simulink model "twotanks_analitico"  (R2017a)
settings: Solver=FixedStepAuto  StartTime=0.0  StopTime=150  FixedStep=0.1  RelTol=1e-3
values from neighbouring files (symbols this model uses):
  H1 = (H1+H1')/2    [MPC_RODAR_PRIMEIRO.m]
  H2 = (H2+H2')/2    [MPC_RODAR_PRIMEIRO.m]
  Phi1 = [Phi1; sysi1.C*sysi1.A^(k)]    [MPC_RODAR_PRIMEIRO.m]
  Phi2 = [Phi2; sysi2.C*sysi2.A^(k)]    [MPC_RODAR_PRIMEIRO.m]
  Q1 = diag(repmat(q,1,Hp))    [MPC_RODAR_PRIMEIRO.m]
  Q2 = diag(repmat(q,1,Hp))    [MPC_RODAR_PRIMEIRO.m]
  Theta1 = [Theta1 aux1]    [MPC_RODAR_PRIMEIRO.m]
  Theta2 = [Theta2 aux2]    [MPC_RODAR_PRIMEIRO.m]
  Vd = 0.00001*eye(nx)    [MPC_RODAR_PRIMEIRO.m]
  Vn = 0.00001*eye(ny)    [MPC_RODAR_PRIMEIRO.m]
undefined symbols (not defined in the file or in its folder): sysi1, sysi2
libraries: simulink x2
settings Model: Creator=raonymaiafontes  LastModifiedBy=aguia
settings SolverCC: ZeroCrossAlgorithm=Adaptive
settings DebuggingCC: MaxConsecutiveZCsMsg=none

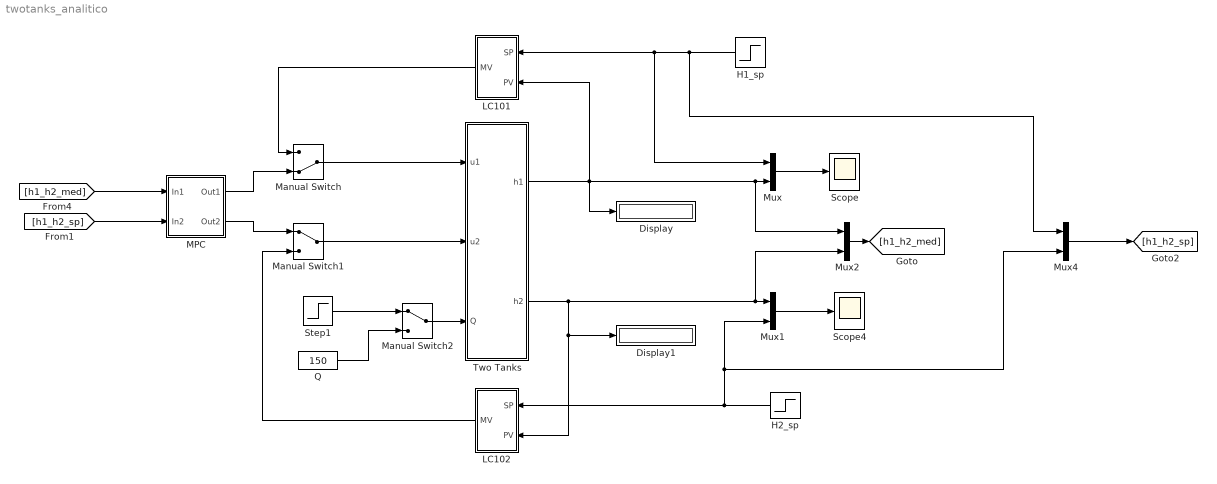
== system twotanks_analitico ==
  Display : Display
  Display1 : Display
  H1_sp : Step  Time=120  Before=0.65  After=0.35  SampleTime=0
  H2_sp : Step  Time=20  Before=0.28  After=0.678  SampleTime=0
  LC101 : Subsystem
  LC102 : Subsystem
  MPC : Subsystem
  Manual Switch : ManualSwitch  CurrentSetting=0
  Manual Switch1 : ManualSwitch
  Manual Switch2 : ManualSwitch
  Mux{,1..2,4} (4 alike) : Mux  Inputs=2
  Q : Constant  Value=150
  Scope : Scope
  Scope4 : Scope
  Step1 : Step  Time=70  Before=150  After=30  SampleTime=0
  Two Tanks : Subsystem
  wires:
  Manual Switch/1 -> Two Tanks/1(u1)
  LC101/1(MV) -> Manual Switch/1
  Manual Switch1/1 -> Two Tanks/2(u2)
  LC102/1(MV) -> Manual Switch1/2
  Manual Switch2/1 -> Two Tanks/3(Q)
  Step1/1 -> Manual Switch2/1
  Q/1 -> Manual Switch2/2
  Mux/1 -> Scope/1
  Mux1/1 -> Scope4/1
  Mux2/1 -> [h1_h2_med]
  Mux4/1 -> [h1_h2_sp]
  Two Tanks/1(h1) -> Mux2/1, Mux/2, LC101/2(PV), Display/1
  Two Tanks/2(h2) -> LC102/2(PV), Display1/1, Mux2/2, Mux1/1
  H2_sp/1 -> Mux4/2, Mux1/2, LC102/1(SP)
  H1_sp/1 -> Mux4/1, Mux/1, LC101/1(SP)
  [h1_h2_med] -> MPC/1(In1)
  [h1_h2_sp] -> MPC/2(In2)
  MPC/2(Out2) -> Manual Switch1/1
  MPC/1(Out1) -> Manual Switch/2

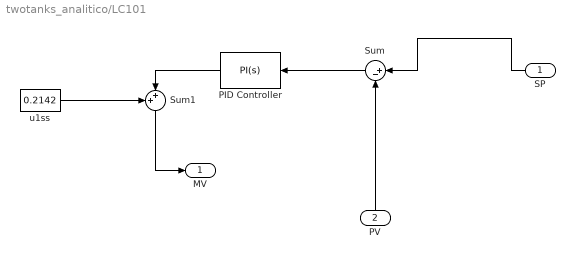
== system twotanks_analitico/LC101 ==
  SP : Inport
  PV : Inport  Port=2
  PID Controller : simulink/Continuous/PID Controller  Controller=PI  TimeDomain=Continuous-time  SampleTime=-1  IntegratorMethod=Forward Euler  FilterMethod=Forward Euler  Form=Ideal  UseFilter=on  ControllerParametersSource=internal  P=-0.667562978885468  I=0.0981942038508327  D=0  N=100  InitialConditionSource=internal  InitialConditionForIntegrator=0  InitialConditionForFilter=0  ExternalReset=none  LimitOutput=on  UpperSaturationLimit=0.7358  LowerSaturationLimit=-0.2042  LinearizeAsGain=on  AntiWindupMode=back-calculation  Kb=1  TrackingMode=off  Kt=1  PParamMin=[]  PParamMax=[]  IParamMin=[]  IParamMax=[]  DParamMin=[]  DParamMax=[]  NParamMin=[]  NParamMax=[]  KbParamMin=[]  KbParamMax=[]  KtParamMin=[]  KtParamMax=[]  POutMin=[]  POutMax=[]  IOutMin=[]  IOutMax=[]  DOutMin=[]  DOutMax=[]  NOutMin=[]  NOutMax=[]  KbOutMin=[]  KbOutMax=[]  KtOutMin=[]  KtOutMax=[]  IntegratorOutMin=[]  IntegratorOutMax=[]  FilterOutMin=[]  FilterOutMax=[]  SumOutMin=[]  SumOutMax=[]  SumI1OutMin=[]  SumI1OutMax=[]  SumI2OutMin=[]  SumI2OutMax=[]  SumI3OutMin=[]  SumI3OutMax=[]  SumDOutMin=[]  SumDOutMax=[]  SaturationOutMin=[]  SaturationOutMax=[]  IntegratorContinuousStateAttributes=''  IntegratorStateMustResolveToSignalObject=off  IntegratorRTWStateStorageClass=Auto  FilterContinuousStateAttributes=''  FilterStateMustResolveToSignalObject=off  FilterRTWStateStorageClass=Auto  DifferentiatorICPrevScaledInput=0  DifferentiatorOutMin=[]  DifferentiatorOutMax=[]  InitialConditionSetting=State (most efficient)
  Sum : Sum  Inputs=|+-
  Sum1 : Sum  Inputs=++|
  u1ss : Constant  Value=0.2142
  MV : Outport
  wires:
  Sum1/1 -> MV/1
  PV/1 -> Sum/2
  PID Controller/1 -> Sum1/2
  SP/1 -> Sum/1
  u1ss/1 -> Sum1/1
  Sum/1 -> PID Controller/1

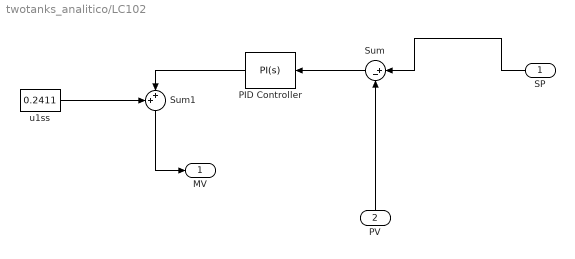
== system twotanks_analitico/LC102 ==
  SP : Inport
  PV : Inport  Port=2
  PID Controller : simulink/Continuous/PID Controller  Controller=PI  TimeDomain=Continuous-time  SampleTime=-1  IntegratorMethod=Forward Euler  FilterMethod=Forward Euler  Form=Ideal  UseFilter=on  ControllerParametersSource=internal  P=-0.11544378631374  I=6.6123973931149  D=0  N=100  InitialConditionSource=internal  InitialConditionForIntegrator=0  InitialConditionForFilter=0  ExternalReset=none  LimitOutput=on  UpperSaturationLimit=0.95-0.2411  LowerSaturationLimit=0.01-0.2411  LinearizeAsGain=on  AntiWindupMode=back-calculation  Kb=1  TrackingMode=off  Kt=1  PParamMin=[]  PParamMax=[]  IParamMin=[]  IParamMax=[]  DParamMin=[]  DParamMax=[]  NParamMin=[]  NParamMax=[]  KbParamMin=[]  KbParamMax=[]  KtParamMin=[]  KtParamMax=[]  POutMin=[]  POutMax=[]  IOutMin=[]  IOutMax=[]  DOutMin=[]  DOutMax=[]  NOutMin=[]  NOutMax=[]  KbOutMin=[]  KbOutMax=[]  KtOutMin=[]  KtOutMax=[]  IntegratorOutMin=[]  IntegratorOutMax=[]  FilterOutMin=[]  FilterOutMax=[]  SumOutMin=[]  SumOutMax=[]  SumI1OutMin=[]  SumI1OutMax=[]  SumI2OutMin=[]  SumI2OutMax=[]  SumI3OutMin=[]  SumI3OutMax=[]  SumDOutMin=[]  SumDOutMax=[]  SaturationOutMin=[]  SaturationOutMax=[]  IntegratorContinuousStateAttributes=''  IntegratorStateMustResolveToSignalObject=off  IntegratorRTWStateStorageClass=Auto  FilterContinuousStateAttributes=''  FilterStateMustResolveToSignalObject=off  FilterRTWStateStorageClass=Auto  DifferentiatorICPrevScaledInput=0  DifferentiatorOutMin=[]  DifferentiatorOutMax=[]  InitialConditionSetting=State (most efficient)
  Sum : Sum  Inputs=|+-
  Sum1 : Sum  Inputs=++|
  u1ss : Constant  Value=0.2411
  MV : Outport
  wires:
  Sum/1 -> PID Controller/1
  u1ss/1 -> Sum1/1
  SP/1 -> Sum/1
  PID Controller/1 -> Sum1/2
  PV/1 -> Sum/2
  Sum1/1 -> MV/1

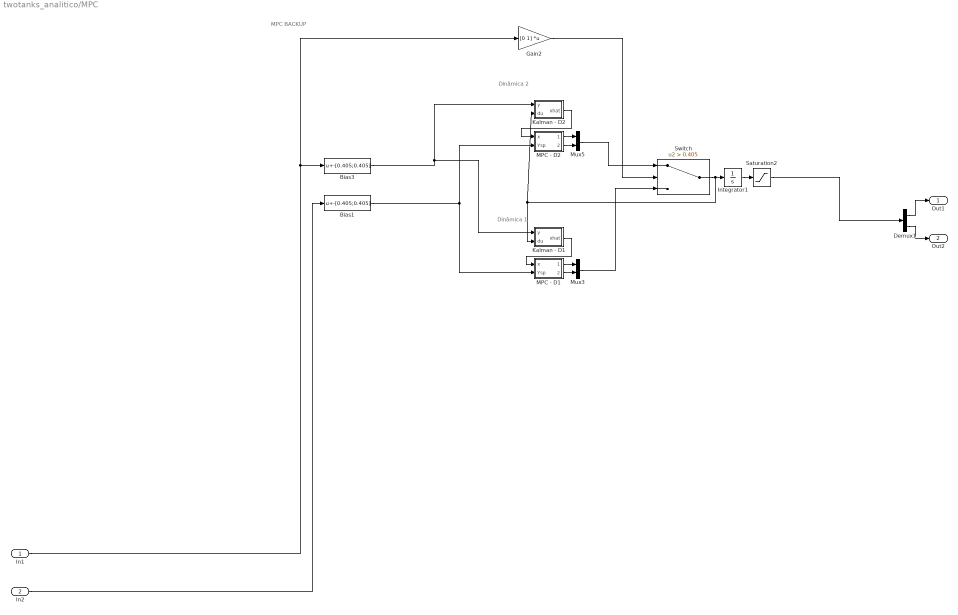
== system twotanks_analitico/MPC ==
  note: MPC BACKUP
  note: Dinâmica 2
  note: Dinâmica 1
  In1 : Inport
  In2 : Inport  Port=2
  Bias1 : Bias  Bias=-[0.405;0.405]
  Bias3 : Bias  Bias=-[0.405;0.405]
  Demux1 : Demux  Outputs=2
  Gain2 : Gain  Gain=[0 1]  Multiplication=Matrix(K*u)
  Integrator1 : Integrator  InitialCondition=[0.2142;0.2411]
  Kalman - D1 : Subsystem
  Kalman - D2 : Subsystem
  MPC - D1 : Subsystem
  MPC - D2 : Subsystem
  Mux3 : Mux  Inputs=2
  Mux5 : Mux  Inputs=2
  Saturation2 : Saturate  UpperLimit=0.95  LowerLimit=0.01
  Switch : Switch  Criteria=u2 > Threshold  Threshold=0.405
  Out1 : Outport
  Out2 : Outport  Port=2
  wires:
  MPC - D1/1(du1) -> Mux3/1
  MPC - D1/2(du2) -> Mux3/2
  MPC - D2/1(du1) -> Mux5/1
  MPC - D2/2(du2) -> Mux5/2
  Bias3/1 -> Kalman - D1/1(y), Kalman - D2/1(y)
  Bias1/1 -> MPC - D1/2(Ysp), MPC - D2/2(Ysp)
  Gain2/1 -> Switch/2
  Integrator1/1 -> Saturation2/1
  Switch/1 -> Integrator1/1, Kalman - D1/2(du), Kalman - D2/2(du)
  Kalman - D1/1(xhat) -> MPC - D1/1(x)
  Kalman - D2/1(xhat) -> MPC - D2/1(x)
  Mux3/1 -> Switch/3
  Mux5/1 -> Switch/1
  In1/1 -> Gain2/1, Bias3/1
  In2/1 -> Bias1/1
  Demux1/1 -> Out1/1
  Demux1/2 -> Out2/1
  Saturation2/1 -> Demux1/1

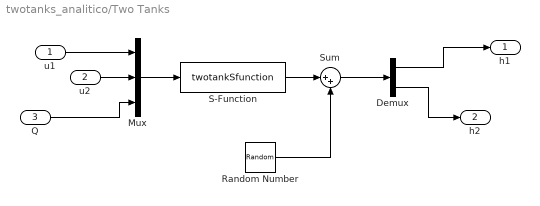
== system twotanks_analitico/Two Tanks ==
  u1 : Inport
  u2 : Inport  Port=2
  Q : Inport  Port=3
  Demux : Demux  Outputs=2
  Mux : Mux  Inputs=3
  Random Number : RandomNumber  Variance=1e-5  SampleTime=0.1
  S-Function : S-Function  FunctionName=twotankSfunction  SFunctionDeploymentMode=off  EnableBusSupport=off
  Sum : Sum  Inputs=|++
  h1 : Outport
  h2 : Outport  Port=2
  wires:
  u2/1 -> Mux/2
  Q/1 -> Mux/3
  Demux/2 -> h2/1
  u1/1 -> Mux/1
  Demux/1 -> h1/1
  Mux/1 -> S-Function/1
  S-Function/1 -> Sum/1
  Sum/1 -> Demux/1
  Random Number/1 -> Sum/2

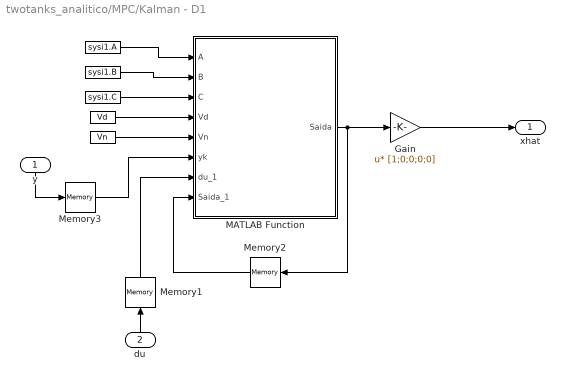
== system twotanks_analitico/MPC/Kalman - D1 ==
  y : Inport
  du : Inport  Port=2
  " " : Constant  Value=sysi1.A
  " " : Constant  Value=sysi1.B
  " " : Constant  Value=sysi1.C
  " " : Constant  Value=Vd
  " " : Constant  Value=Vn
  Gain : Gain  Gain=[1;0;0;0;0]  Multiplication=Matrix(u*K)
  MATLAB Function : MATLAB Function  TreatAsAtomicUnit=on
  Memory1 : Memory  X0=[0;0]
  Memory2 : Memory  X0=[zeros(4,1), Vd]
  Memory3 : Memory  X0=[0;0]
  xhat : Outport
  wires:
  y/1 -> Memory3/1
  du/1 -> Memory1/1
  MATLAB Function/1(Saida) -> Gain/1, Memory2/1
  Gain/1 -> xhat/1
  Memory2/1 -> MATLAB Function/8(Saida_1)
  Memory3/1 -> MATLAB Function/6(yk)
  Memory1/1 -> MATLAB Function/7(du_1)
  " "/1 -> MATLAB Function/2(B)
  " "/1 -> MATLAB Function/3(C)
  " "/1 -> MATLAB Function/5(Vn)
  " "/1 -> MATLAB Function/1(A)
  " "/1 -> MATLAB Function/4(Vd)

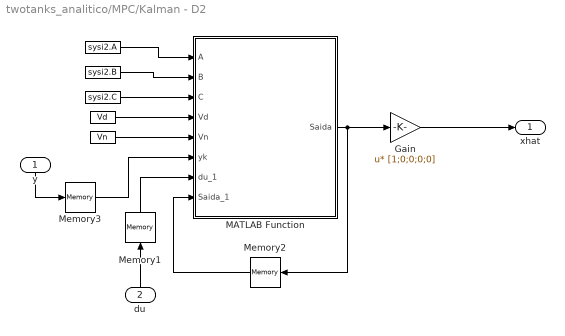
== system twotanks_analitico/MPC/Kalman - D2 ==
  y : Inport
  du : Inport  Port=2
  " " : Constant  Value=sysi2.A
  " " : Constant  Value=sysi2.B
  " " : Constant  Value=sysi2.C
  " " : Constant  Value=Vd
  " " : Constant  Value=Vn
  Gain : Gain  Gain=[1;0;0;0;0]  Multiplication=Matrix(u*K)
  MATLAB Function : MATLAB Function  TreatAsAtomicUnit=on
  Memory1 : Memory  X0=[0;0]
  Memory2 : Memory  X0=[zeros(4,1), Vd]
  Memory3 : Memory  X0=[0;0]
  xhat : Outport
  wires:
  " "/1 -> MATLAB Function/4(Vd)
  " "/1 -> MATLAB Function/1(A)
  " "/1 -> MATLAB Function/5(Vn)
  " "/1 -> MATLAB Function/3(C)
  " "/1 -> MATLAB Function/2(B)
  Memory1/1 -> MATLAB Function/7(du_1)
  Memory3/1 -> MATLAB Function/6(yk)
  Memory2/1 -> MATLAB Function/8(Saida_1)
  Gain/1 -> xhat/1
  MATLAB Function/1(Saida) -> Memory2/1, Gain/1
  du/1 -> Memory1/1
  y/1 -> Memory3/1

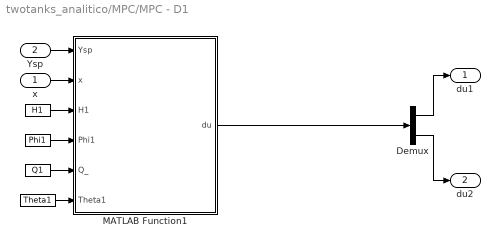
== system twotanks_analitico/MPC/MPC - D1 ==
  x : Inport
  Ysp : Inport  Port=2
  " " : Constant  Value=H1
  "  " : Constant  Value=Q1
  "   " : Constant  Value=Phi1
  "    " : Constant  Value=Theta1
  Demux : Demux  Outputs=2
  MATLAB Function1 : MATLAB Function  TreatAsAtomicUnit=on
  du1 : Outport
  du2 : Outport  Port=2
  wires:
  MATLAB Function1/1(du) -> Demux/1
  "  "/1 -> MATLAB Function1/5(Q_)
  "    "/1 -> MATLAB Function1/6(Theta1)
  " "/1 -> MATLAB Function1/3(H1)
  "   "/1 -> MATLAB Function1/4(Phi1)
  Ysp/1 -> MATLAB Function1/1(Ysp)
  x/1 -> MATLAB Function1/2(x)
  Demux/1 -> du1/1
  Demux/2 -> du2/1

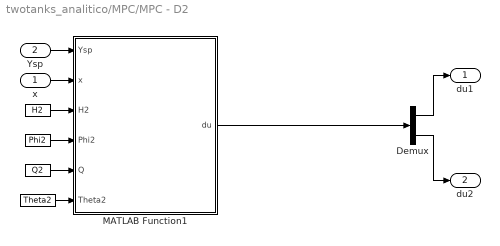
== system twotanks_analitico/MPC/MPC - D2 ==
  x : Inport
  Ysp : Inport  Port=2
  " " : Constant  Value=H2
  "  " : Constant  Value=Q2
  "   " : Constant  Value=Phi2
  "    " : Constant  Value=Theta2
  Demux : Demux  Outputs=2
  MATLAB Function1 : MATLAB Function  TreatAsAtomicUnit=on
  du1 : Outport
  du2 : Outport  Port=2
  wires:
  Demux/2 -> du2/1
  Demux/1 -> du1/1
  x/1 -> MATLAB Function1/2(x)
  Ysp/1 -> MATLAB Function1/1(Ysp)
  "   "/1 -> MATLAB Function1/4(Phi2)
  " "/1 -> MATLAB Function1/3(H2)
  "    "/1 -> MATLAB Function1/6(Theta2)
  "  "/1 -> MATLAB Function1/5(Q)
  MATLAB Function1/1(du) -> Demux/1

== matlab function twotanks_analitico/MPC/Kalman - D1/MATLAB Function ==
  data: A input; B input; C input; Vd input; Vn input; yk input; du_1 input; Saida_1 input; Saida output
function Saida = fcn(A, B, C, Vd, Vn, yk, du_1, Saida_1 )
    nx = length(A);
    xmk = Saida_1(:,1);
    P = Saida_1(:,2:end);
    % Filtro de kalman - predicao
    xmk = A*xmk + B*(du_1);
    ymk = C*xmk;
    P = A*P*A' + Vd;
    % Filtro de Kalman - correcao
    K = P*C'/(C*P*C' + Vn);
    xmk = xmk + K*(yk - ymk);
    P = (eye(nx) - K*C)*P;
    Saida = [xmk,P];

== matlab function twotanks_analitico/MPC/MPC - D1/MATLAB Function1 ==
  data: Ysp input; x input; H1 input; Phi1 input; Q_ input; Theta1 input; du output
function du = fcn(Ysp, x, H1, Phi1, Q_, Theta1 )
Ysp = repmat(Ysp,(length(Q_)/length(Ysp)),1);   
cf = (Phi1*x)'*Q_*Theta1 - Ysp'*Q_*Theta1;
du_ = (-H1^-1*cf');
du = du_(1:2,1);

== matlab function twotanks_analitico/MPC/MPC - D2/MATLAB Function1 ==
  data: Ysp input; x input; H2 input; Phi2 input; Q input; Theta2 input; du output
function du = fcn(Ysp, x, H2, Phi2, Q, Theta2 )
Ysp = repmat(Ysp,(length(Q)/length(Ysp)),1);   
cf = (Phi2*x)'*Q*Theta2 - Ysp'*Q*Theta2;
du_ = (-H2^-1*cf');
du = du_(1:2,1);

== matlab function twotanks_analitico/MPC/Kalman - D2/MATLAB Function ==
  data: A input; B input; C input; Vd input; Vn input; yk input; du_1 input; Saida_1 input; Saida output
function Saida = fcn(A, B, C, Vd, Vn, yk, du_1, Saida_1 )
    nx = length(A);
    xmk = Saida_1(:,1);
    P = Saida_1(:,2:end);
    % Filtro de kalman - predicao
    xmk = (A)*xmk + B*(du_1);
    ymk = C*xmk;
    P = A*P*A' + Vd;
    % Filtro de Kalman - correcao
    K = P*C'/(C*P*C' + Vn);
    xmk = xmk + K*(yk - ymk);
    P = (eye(nx) - K*C)*P;
    Saida = [xmk,P];
